simulink library "rewardLibrary"  (R2022b)
settings: Solver=VariableStepAuto  StartTime=0.0  StopTime=10.0  RelTol=1e-3
values from neighbouring files (symbols this model uses):
  accel_vec = (-4:0.5:4)'    [setUpModel.m]
  Ts = 0.1    [setUpMPC.m]
  TsRL = Ts    [setUpRLEnv.m]
  vel_vec = 0:2:20    [setUpModel.m]
undefined symbols (not defined in the file or in its folder): A, B, C, curvature1, D, D_default, DiscIntNeverNeededParam, E, F, gradbp1, k_sigmoid, steer_lim, t_gap, v_set, x_colpen, y_colpen, Z_colpen
libraries: simulink x379, $bdroot x2, mpcadaslib x1
(part 4 of 9)

== system rewardLibrary/Obs // Reward 2-3/Subsystem2 ==
  v_ego : Inport
  e1 : Inport  Port=2
  e2 : Inport  Port=3
  AND : Logic  IconShape=distinctive  AllPortsSameDT=off  OutDataTypeStr=boolean
  Abs : Abs  SaturateOnIntegerOverflow=off
  Abs1 : Abs  SaturateOnIntegerOverflow=off
  Lateral deviation : simulink/Logic and Bit Operations/Compare To Constant  relop=>  const=8  OutDataTypeStr=boolean
  Logical Operator : Logic  Operator=OR  AllPortsSameDT=off  OutDataTypeStr=boolean
  R2D : Gain  Gain=180/pi
  Relative yaw angle : simulink/Logic and Bit Operations/Compare To Constant  relop=>  const=60  OutDataTypeStr=boolean
  Velocity : simulink/Logic and Bit Operations/Compare To Constant  relop=<  const=0.5  OutDataTypeStr=boolean
  Velocity1 : simulink/Logic and Bit Operations/Compare To Constant  relop=<  const=10  OutDataTypeStr=boolean
  isDone : Outport  VectorParamsAs1DForOutWhenUnconnected=off
  spinTurn : Outport  Port=2  VectorParamsAs1DForOutWhenUnconnected=off
  wires:
  Velocity/1 -> Logical Operator/1
  Logical Operator/1 -> isDone/1
  v_ego/1 -> Velocity1/1, Velocity/1
  Abs/1 -> Lateral deviation/1
  Lateral deviation/1 -> Logical Operator/2
  e1/1 -> Abs/1
  Velocity1/1 -> AND/1
  e2/1 -> Abs1/1
  Abs1/1 -> R2D/1
  R2D/1 -> Relative yaw angle/1
  Relative yaw angle/1 -> AND/2
  AND/1 -> spinTurn/1

== system rewardLibrary/Obs // Reward 2-4/Subsystem ==
  v_ego : Inport
  v_ref : Inport  Port=2
  e1 : Inport  Port=3
  e2 : Inport  Port=4
  e1dot : Inport  Port=5
  e2dot : Inport  Port=6
  Add : Sum  Inputs=+-
  Discrete-Time Integrator1 : DiscreteIntegrator  SampleTime=-1  ICPrevOutput=DiscIntNeverNeededParam  ICPrevScaledInput=DiscIntNeverNeededParam
  Discrete-Time Integrator2 : DiscreteIntegrator  SampleTime=-1  ICPrevOutput=DiscIntNeverNeededParam  ICPrevScaledInput=DiscIntNeverNeededParam
  Discrete-Time Integrator3 : DiscreteIntegrator  SampleTime=-1  ICPrevOutput=DiscIntNeverNeededParam  ICPrevScaledInput=DiscIntNeverNeededParam
  Lateral deviation : Scope
  Mux : Mux  Inputs=9
  obs : Outport  VectorParamsAs1DForOutWhenUnconnected=off
  v_err : Outport  Port=2  VectorParamsAs1DForOutWhenUnconnected=off
  wires:
  Add/1 -> v_err/1, Mux/2, Discrete-Time Integrator1/1
  Discrete-Time Integrator3/1 -> Mux/6  "integral_error"
  v_ego/1 -> Add/2, Mux/3
  e1/1 -> Lateral deviation/1, Mux/5, Discrete-Time Integrator2/1
  Discrete-Time Integrator1/1 -> Mux/1  "integral_error"
  e2/1 -> Mux/7, Discrete-Time Integrator3/1
  Discrete-Time Integrator2/1 -> Mux/4  "integral_error"
  Mux/1 -> obs/1
  e1dot/1 -> Mux/8
  e2dot/1 -> Mux/9
  v_ref/1 -> Add/1  "d_rel"

== system rewardLibrary/Obs // Reward 2-4/Subsystem1 ==
  steer : Inport
  e1 : Inport  Port=2
  v_err : Inport  Port=3
  accel : Inport  Port=4
  Compare To Constant : simulink/Logic and Bit Operations/Compare To Constant  relop=<  const=1  OutDataTypeStr=boolean
  Compare To Constant1 : simulink/Logic and Bit Operations/Compare To Constant  relop=<  const=4  OutDataTypeStr=boolean
  Digital Clock : DigitalClock  Commented=on  SampleTime=Ts
  Gain : Gain  Gain=100
  Gain1 : Gain
  Gain2 : Gain  Gain=500
  Gain3 : Gain  Gain=2
  Gain4 : Gain  Gain=1e-3
  Gain5 : Gain  Commented=on  Gain=1/10
  Gain6 : Gain  Gain=100
  Gain7 : Gain  Gain=10
  Math Function2 : Math  Operator=square  SignedPower=on
  Square : Math  Operator=square  SignedPower=on
  Square2 : Math  Operator=square  SignedPower=on
  Square5 : Math  Operator=square  SignedPower=on
  Sum : Sum  Inputs=----
  Sum1 : Sum  Inputs=++++
  Unit Delay : UnitDelay  SampleTime=-1  HasFrameUpgradeWarning=on
  Unit Delay1 : UnitDelay  SampleTime=-1  HasFrameUpgradeWarning=on
  reward : Outport  VectorParamsAs1DForOutWhenUnconnected=off
  wires:
  v_err/1 -> Square5/1
  Square/1 -> Compare To Constant1/1, Gain/1
  Sum1/1 -> reward/1
  accel/1 -> Unit Delay1/1
  Gain6/1 -> Sum/4
  Compare To Constant/1 -> Gain1/1
  Math Function2/1 -> Gain6/1
  Gain3/1 -> Sum1/1
  Compare To Constant1/1 -> Gain3/1
  Square2/1 -> Gain2/1
  Gain7/1 -> Sum/3
  Unit Delay1/1 -> Math Function2/1
  Gain1/1 -> Sum1/3
  steer/1 -> Unit Delay/1
  Gain2/1 -> Sum/2
  Sum/1 -> Gain4/1
  Unit Delay/1 -> Square2/1
  Square5/1 -> Compare To Constant/1, Gain7/1
  Gain/1 -> Sum/1
  Gain4/1 -> Sum1/2
  e1/1 -> Square/1
  Digital Clock/1 -> Gain5/1
  Gain5/1 -> Sum1/4

== system rewardLibrary/Obs // Reward 2-4/Subsystem2 ==
  v_ego : Inport
  e1 : Inport  Port=2
  e2 : Inport  Port=3
  AND : Logic  IconShape=distinctive  AllPortsSameDT=off  OutDataTypeStr=boolean
  Abs : Abs  SaturateOnIntegerOverflow=off
  Abs1 : Abs  SaturateOnIntegerOverflow=off
  Lateral deviation : simulink/Logic and Bit Operations/Compare To Constant  relop=>  const=8  OutDataTypeStr=boolean
  Logical Operator : Logic  Operator=OR  AllPortsSameDT=off  OutDataTypeStr=boolean
  R2D : Gain  Gain=180/pi
  Relative yaw angle : simulink/Logic and Bit Operations/Compare To Constant  relop=>  const=60  OutDataTypeStr=boolean
  Velocity : simulink/Logic and Bit Operations/Compare To Constant  relop=<  const=0.5  OutDataTypeStr=boolean
  Velocity1 : simulink/Logic and Bit Operations/Compare To Constant  relop=<  const=10  OutDataTypeStr=boolean
  isDone : Outport  VectorParamsAs1DForOutWhenUnconnected=off
  spinTurn : Outport  Port=2  VectorParamsAs1DForOutWhenUnconnected=off
  wires:
  Velocity/1 -> Logical Operator/1
  Logical Operator/1 -> isDone/1
  v_ego/1 -> Velocity1/1, Velocity/1
  Abs/1 -> Lateral deviation/1
  Lateral deviation/1 -> Logical Operator/2
  e1/1 -> Abs/1
  Velocity1/1 -> AND/1
  e2/1 -> Abs1/1
  Abs1/1 -> R2D/1
  R2D/1 -> Relative yaw angle/1
  Relative yaw angle/1 -> AND/2
  AND/1 -> spinTurn/1

== system rewardLibrary/Obs // Reward 2-5/Subsystem ==
  v_ego : Inport
  v_ref : Inport  Port=2
  e1 : Inport  Port=3
  e2 : Inport  Port=4
  e1dot : Inport  Port=5
  e2dot : Inport  Port=6
  Add : Sum  Inputs=+-
  Discrete-Time Integrator1 : DiscreteIntegrator  SampleTime=-1  ICPrevOutput=DiscIntNeverNeededParam  ICPrevScaledInput=DiscIntNeverNeededParam
  Discrete-Time Integrator2 : DiscreteIntegrator  SampleTime=-1  ICPrevOutput=DiscIntNeverNeededParam  ICPrevScaledInput=DiscIntNeverNeededParam
  Discrete-Time Integrator3 : DiscreteIntegrator  SampleTime=-1  ICPrevOutput=DiscIntNeverNeededParam  ICPrevScaledInput=DiscIntNeverNeededParam
  Lateral deviation : Scope
  Mux : Mux  Inputs=9
  obs : Outport  VectorParamsAs1DForOutWhenUnconnected=off
  v_err : Outport  Port=2  VectorParamsAs1DForOutWhenUnconnected=off
  wires:
  Add/1 -> v_err/1, Mux/2, Discrete-Time Integrator1/1
  Discrete-Time Integrator3/1 -> Mux/6  "integral_error"
  v_ego/1 -> Add/2, Mux/3
  e1/1 -> Lateral deviation/1, Mux/5, Discrete-Time Integrator2/1
  Discrete-Time Integrator1/1 -> Mux/1  "integral_error"
  e2/1 -> Mux/7, Discrete-Time Integrator3/1
  Discrete-Time Integrator2/1 -> Mux/4  "integral_error"
  Mux/1 -> obs/1
  e1dot/1 -> Mux/8
  e2dot/1 -> Mux/9
  v_ref/1 -> Add/1  "d_rel"

== system rewardLibrary/Obs // Reward 2-5/Subsystem1 ==
  steer : Inport
  e1 : Inport  Port=2
  v_err : Inport  Port=3
  accel : Inport  Port=4
  Compare To Constant : simulink/Logic and Bit Operations/Compare To Constant  relop=<  const=1  OutDataTypeStr=boolean
  Compare To Constant1 : simulink/Logic and Bit Operations/Compare To Constant  relop=<  const=4  OutDataTypeStr=boolean
  Digital Clock : DigitalClock  Commented=on  SampleTime=Ts
  Gain : Gain  Gain=100
  Gain1 : Gain
  Gain2 : Gain  Gain=500
  Gain3 : Gain  Gain=2
  Gain4 : Gain  Gain=1e-3
  Gain5 : Gain  Commented=on  Gain=1/10
  Gain6 : Gain  Gain=100
  Gain7 : Gain  Gain=10
  Math Function2 : Math  Operator=square  SignedPower=on
  Square : Math  Operator=square  SignedPower=on
  Square2 : Math  Operator=square  SignedPower=on
  Square5 : Math  Operator=square  SignedPower=on
  Sum : Sum  Inputs=----
  Sum1 : Sum  Inputs=++++
  Unit Delay : UnitDelay  SampleTime=-1  HasFrameUpgradeWarning=on
  Unit Delay1 : UnitDelay  SampleTime=-1  HasFrameUpgradeWarning=on
  reward : Outport  VectorParamsAs1DForOutWhenUnconnected=off
  wires:
  v_err/1 -> Square5/1
  Square/1 -> Compare To Constant1/1, Gain/1
  Sum1/1 -> reward/1
  accel/1 -> Unit Delay1/1
  Gain6/1 -> Sum/4
  Compare To Constant/1 -> Gain1/1
  Math Function2/1 -> Gain6/1
  Gain3/1 -> Sum1/1
  Compare To Constant1/1 -> Gain3/1
  Square2/1 -> Gain2/1
  Gain7/1 -> Sum/3
  Unit Delay1/1 -> Math Function2/1
  Gain1/1 -> Sum1/3
  steer/1 -> Unit Delay/1
  Gain2/1 -> Sum/2
  Sum/1 -> Gain4/1
  Unit Delay/1 -> Square2/1
  Square5/1 -> Compare To Constant/1, Gain7/1
  Gain/1 -> Sum/1
  Gain4/1 -> Sum1/2
  e1/1 -> Square/1
  Digital Clock/1 -> Gain5/1
  Gain5/1 -> Sum1/4

== system rewardLibrary/Obs // Reward 2-5/Subsystem2 ==
  v_ego : Inport
  e1 : Inport  Port=2
  e2 : Inport  Port=3
  AND : Logic  IconShape=distinctive  AllPortsSameDT=off  OutDataTypeStr=boolean
  Abs : Abs  SaturateOnIntegerOverflow=off
  Abs1 : Abs  SaturateOnIntegerOverflow=off
  Lateral deviation : simulink/Logic and Bit Operations/Compare To Constant  relop=>  const=8  OutDataTypeStr=boolean
  Logical Operator : Logic  Operator=OR  AllPortsSameDT=off  OutDataTypeStr=boolean
  R2D : Gain  Gain=180/pi
  Relative yaw angle : simulink/Logic and Bit Operations/Compare To Constant  relop=>  const=60  OutDataTypeStr=boolean
  Velocity : simulink/Logic and Bit Operations/Compare To Constant  relop=<  const=2.5  OutDataTypeStr=boolean
  Velocity1 : simulink/Logic and Bit Operations/Compare To Constant  relop=<  const=10  OutDataTypeStr=boolean
  isDone : Outport  VectorParamsAs1DForOutWhenUnconnected=off
  spinTurn : Outport  Port=2  VectorParamsAs1DForOutWhenUnconnected=off
  wires:
  Velocity/1 -> Logical Operator/1
  Logical Operator/1 -> isDone/1
  v_ego/1 -> Velocity1/1, Velocity/1
  Abs/1 -> Lateral deviation/1
  Lateral deviation/1 -> Logical Operator/2
  e1/1 -> Abs/1
  Velocity1/1 -> AND/1
  e2/1 -> Abs1/1
  Abs1/1 -> R2D/1
  R2D/1 -> Relative yaw angle/1
  Relative yaw angle/1 -> AND/2
  AND/1 -> spinTurn/1

== system rewardLibrary/Obs // Reward 2-6/Subsystem ==
  v_ego : Inport
  v_ref : Inport  Port=2
  e1 : Inport  Port=3
  e2 : Inport  Port=4
  e1dot : Inport  Port=5
  e2dot : Inport  Port=6
  Add : Sum  Inputs=+-
  Discrete-Time Integrator1 : DiscreteIntegrator  SampleTime=-1  ICPrevOutput=DiscIntNeverNeededParam  ICPrevScaledInput=DiscIntNeverNeededParam
  Discrete-Time Integrator2 : DiscreteIntegrator  SampleTime=-1  ICPrevOutput=DiscIntNeverNeededParam  ICPrevScaledInput=DiscIntNeverNeededParam
  Discrete-Time Integrator3 : DiscreteIntegrator  SampleTime=-1  ICPrevOutput=DiscIntNeverNeededParam  ICPrevScaledInput=DiscIntNeverNeededParam
  Lateral deviation : Scope
  Mux : Mux  Inputs=9
  obs : Outport  VectorParamsAs1DForOutWhenUnconnected=off
  v_err : Outport  Port=2  VectorParamsAs1DForOutWhenUnconnected=off
  wires:
  Add/1 -> v_err/1, Mux/2, Discrete-Time Integrator1/1
  Discrete-Time Integrator3/1 -> Mux/6  "integral_error"
  v_ego/1 -> Add/2, Mux/3
  e1/1 -> Lateral deviation/1, Mux/5, Discrete-Time Integrator2/1
  Discrete-Time Integrator1/1 -> Mux/1  "integral_error"
  e2/1 -> Mux/7, Discrete-Time Integrator3/1
  Discrete-Time Integrator2/1 -> Mux/4  "integral_error"
  Mux/1 -> obs/1
  e1dot/1 -> Mux/8
  e2dot/1 -> Mux/9
  v_ref/1 -> Add/1  "d_rel"

== system rewardLibrary/Obs // Reward 2-6/Subsystem1 ==
  steer : Inport
  e1 : Inport  Port=2
  v_err : Inport  Port=3
  accel : Inport  Port=4
  Compare To Constant : simulink/Logic and Bit Operations/Compare To Constant  relop=<  const=1  OutDataTypeStr=boolean
  Compare To Constant1 : simulink/Logic and Bit Operations/Compare To Constant  relop=<  const=4  OutDataTypeStr=boolean
  Digital Clock : DigitalClock  Commented=on  SampleTime=Ts
  Gain : Gain  Gain=100
  Gain1 : Gain
  Gain2 : Gain  Gain=500
  Gain3 : Gain  Gain=2
  Gain4 : Gain  Gain=1e-3
  Gain5 : Gain  Commented=on  Gain=1/10
  Gain6 : Gain  Gain=100
  Gain7 : Gain  Gain=20
  Math Function2 : Math  Operator=square  SignedPower=on
  Square : Math  Operator=square  SignedPower=on
  Square2 : Math  Operator=square  SignedPower=on
  Square5 : Math  Operator=square  SignedPower=on
  Sum : Sum  Inputs=----
  Sum1 : Sum  Inputs=++++
  Unit Delay : UnitDelay  SampleTime=-1  HasFrameUpgradeWarning=on
  Unit Delay1 : UnitDelay  SampleTime=-1  HasFrameUpgradeWarning=on
  reward : Outport  VectorParamsAs1DForOutWhenUnconnected=off
  wires:
  v_err/1 -> Square5/1
  Square/1 -> Compare To Constant1/1, Gain/1
  Sum1/1 -> reward/1
  accel/1 -> Unit Delay1/1
  Gain6/1 -> Sum/4
  Compare To Constant/1 -> Gain1/1
  Math Function2/1 -> Gain6/1
  Gain3/1 -> Sum1/1
  Compare To Constant1/1 -> Gain3/1
  Square2/1 -> Gain2/1
  Gain7/1 -> Sum/3
  Unit Delay1/1 -> Math Function2/1
  Gain1/1 -> Sum1/3
  steer/1 -> Unit Delay/1
  Gain2/1 -> Sum/2
  Sum/1 -> Gain4/1
  Unit Delay/1 -> Square2/1
  Square5/1 -> Compare To Constant/1, Gain7/1
  Gain/1 -> Sum/1
  Gain4/1 -> Sum1/2
  e1/1 -> Square/1
  Digital Clock/1 -> Gain5/1
  Gain5/1 -> Sum1/4

== system rewardLibrary/Obs // Reward 2-6/Subsystem2 ==
  v_ego : Inport
  e1 : Inport  Port=2
  e2 : Inport  Port=3
  AND : Logic  IconShape=distinctive  AllPortsSameDT=off  OutDataTypeStr=boolean
  Abs : Abs  SaturateOnIntegerOverflow=off
  Abs1 : Abs  SaturateOnIntegerOverflow=off
  Lateral deviation : simulink/Logic and Bit Operations/Compare To Constant  relop=>  const=8  OutDataTypeStr=boolean
  Logical Operator : Logic  Operator=OR  AllPortsSameDT=off  OutDataTypeStr=boolean
  R2D : Gain  Gain=180/pi
  Relative yaw angle : simulink/Logic and Bit Operations/Compare To Constant  relop=>  const=60  OutDataTypeStr=boolean
  Velocity : simulink/Logic and Bit Operations/Compare To Constant  relop=<  const=4  OutDataTypeStr=boolean
  Velocity1 : simulink/Logic and Bit Operations/Compare To Constant  relop=<  const=10  OutDataTypeStr=boolean
  isDone : Outport  VectorParamsAs1DForOutWhenUnconnected=off
  spinTurn : Outport  Port=2  VectorParamsAs1DForOutWhenUnconnected=off
  wires:
  Velocity/1 -> Logical Operator/1
  Logical Operator/1 -> isDone/1
  v_ego/1 -> Velocity1/1, Velocity/1
  Abs/1 -> Lateral deviation/1
  Lateral deviation/1 -> Logical Operator/2
  e1/1 -> Abs/1
  Velocity1/1 -> AND/1
  e2/1 -> Abs1/1
  Abs1/1 -> R2D/1
  R2D/1 -> Relative yaw angle/1
  Relative yaw angle/1 -> AND/2
  AND/1 -> spinTurn/1

== system rewardLibrary/Obs // Reward 2-7/Subsystem ==
  v_ego : Inport
  v_ref : Inport  Port=2
  e1 : Inport  Port=3
  e2 : Inport  Port=4
  e1dot : Inport  Port=5
  e2dot : Inport  Port=6
  Add : Sum  Inputs=+-
  Discrete-Time Integrator1 : DiscreteIntegrator  SampleTime=-1  ICPrevOutput=DiscIntNeverNeededParam  ICPrevScaledInput=DiscIntNeverNeededParam
  Discrete-Time Integrator2 : DiscreteIntegrator  SampleTime=-1  ICPrevOutput=DiscIntNeverNeededParam  ICPrevScaledInput=DiscIntNeverNeededParam
  Discrete-Time Integrator3 : DiscreteIntegrator  SampleTime=-1  ICPrevOutput=DiscIntNeverNeededParam  ICPrevScaledInput=DiscIntNeverNeededParam
  Lateral deviation : Scope
  Mux : Mux  Inputs=9
  obs : Outport  VectorParamsAs1DForOutWhenUnconnected=off
  v_err : Outport  Port=2  VectorParamsAs1DForOutWhenUnconnected=off
  wires:
  Add/1 -> v_err/1, Mux/2, Discrete-Time Integrator1/1
  Discrete-Time Integrator3/1 -> Mux/6  "integral_error"
  v_ego/1 -> Add/2, Mux/3
  e1/1 -> Lateral deviation/1, Mux/5, Discrete-Time Integrator2/1
  Discrete-Time Integrator1/1 -> Mux/1  "integral_error"
  e2/1 -> Mux/7, Discrete-Time Integrator3/1
  Discrete-Time Integrator2/1 -> Mux/4  "integral_error"
  Mux/1 -> obs/1
  e1dot/1 -> Mux/8
  e2dot/1 -> Mux/9
  v_ref/1 -> Add/1  "d_rel"

== system rewardLibrary/Obs // Reward 2-7/Subsystem1 ==
  steer : Inport
  e1 : Inport  Port=2
  v_err : Inport  Port=3
  accel : Inport  Port=4
  Compare To Constant : simulink/Logic and Bit Operations/Compare To Constant  relop=<  const=1  OutDataTypeStr=boolean
  Compare To Constant1 : simulink/Logic and Bit Operations/Compare To Constant  relop=<  const=4  OutDataTypeStr=boolean
  Digital Clock : DigitalClock  Commented=on  SampleTime=Ts
  Gain : Gain  Gain=100
  Gain1 : Gain
  Gain2 : Gain  Gain=500
  Gain3 : Gain  Gain=2
  Gain4 : Gain  Gain=1e-3
  Gain5 : Gain  Commented=on  Gain=1/10
  Gain6 : Gain  Gain=100
  Gain7 : Gain  Gain=20
  Math Function2 : Math  Operator=square  SignedPower=on
  Square : Math  Operator=square  SignedPower=on
  Square2 : Math  Operator=square  SignedPower=on
  Square5 : Math  Operator=square  SignedPower=on
  Sum : Sum  Inputs=----
  Sum1 : Sum  Inputs=++++
  Unit Delay : UnitDelay  SampleTime=-1  HasFrameUpgradeWarning=on
  Unit Delay1 : UnitDelay  SampleTime=-1  HasFrameUpgradeWarning=on
  reward : Outport  VectorParamsAs1DForOutWhenUnconnected=off
  wires:
  v_err/1 -> Square5/1
  Square/1 -> Compare To Constant1/1, Gain/1
  Sum1/1 -> reward/1
  accel/1 -> Unit Delay1/1
  Gain6/1 -> Sum/4
  Compare To Constant/1 -> Gain1/1
  Math Function2/1 -> Gain6/1
  Gain3/1 -> Sum1/1
  Compare To Constant1/1 -> Gain3/1
  Square2/1 -> Gain2/1
  Gain7/1 -> Sum/3
  Unit Delay1/1 -> Math Function2/1
  Gain1/1 -> Sum1/3
  steer/1 -> Unit Delay/1
  Gain2/1 -> Sum/2
  Sum/1 -> Gain4/1
  Unit Delay/1 -> Square2/1
  Square5/1 -> Compare To Constant/1, Gain7/1
  Gain/1 -> Sum/1
  Gain4/1 -> Sum1/2
  e1/1 -> Square/1
  Digital Clock/1 -> Gain5/1
  Gain5/1 -> Sum1/4

== system rewardLibrary/Obs // Reward 2-7/Subsystem2 ==
  v_ego : Inport
  e1 : Inport  Port=2
  e2 : Inport  Port=3
  AND : Logic  IconShape=distinctive  AllPortsSameDT=off  OutDataTypeStr=boolean
  Abs : Abs  SaturateOnIntegerOverflow=off
  Abs1 : Abs  SaturateOnIntegerOverflow=off
  Lateral deviation : simulink/Logic and Bit Operations/Compare To Constant  relop=>  const=12  OutDataTypeStr=boolean
  Logical Operator : Logic  Operator=OR  AllPortsSameDT=off  OutDataTypeStr=boolean
  R2D : Gain  Gain=180/pi
  Relative yaw angle : simulink/Logic and Bit Operations/Compare To Constant  relop=>  const=60  OutDataTypeStr=boolean
  Velocity : simulink/Logic and Bit Operations/Compare To Constant  relop=<  const=4  OutDataTypeStr=boolean
  Velocity1 : simulink/Logic and Bit Operations/Compare To Constant  relop=<  const=10  OutDataTypeStr=boolean
  isDone : Outport  VectorParamsAs1DForOutWhenUnconnected=off
  spinTurn : Outport  Port=2  VectorParamsAs1DForOutWhenUnconnected=off
  wires:
  Velocity/1 -> Logical Operator/1
  Logical Operator/1 -> isDone/1
  v_ego/1 -> Velocity1/1, Velocity/1
  Abs/1 -> Lateral deviation/1
  Lateral deviation/1 -> Logical Operator/2
  e1/1 -> Abs/1
  Velocity1/1 -> AND/1
  e2/1 -> Abs1/1
  Abs1/1 -> R2D/1
  R2D/1 -> Relative yaw angle/1
  Relative yaw angle/1 -> AND/2
  AND/1 -> spinTurn/1

== system rewardLibrary/Obs // Reward 2-8/Subsystem ==
  v_ego : Inport
  v_ref : Inport  Port=2
  e1 : Inport  Port=3
  e2 : Inport  Port=4
  e1dot : Inport  Port=5
  e2dot : Inport  Port=6
  Add : Sum  Inputs=+-
  Discrete-Time Integrator1 : DiscreteIntegrator  SampleTime=-1  ICPrevOutput=DiscIntNeverNeededParam  ICPrevScaledInput=DiscIntNeverNeededParam
  Discrete-Time Integrator2 : DiscreteIntegrator  SampleTime=-1  ICPrevOutput=DiscIntNeverNeededParam  ICPrevScaledInput=DiscIntNeverNeededParam
  Discrete-Time Integrator3 : DiscreteIntegrator  SampleTime=-1  ICPrevOutput=DiscIntNeverNeededParam  ICPrevScaledInput=DiscIntNeverNeededParam
  Lateral deviation : Scope
  Mux : Mux  Inputs=9
  obs : Outport  VectorParamsAs1DForOutWhenUnconnected=off
  v_err : Outport  Port=2  VectorParamsAs1DForOutWhenUnconnected=off
  wires:
  Add/1 -> v_err/1, Mux/2, Discrete-Time Integrator1/1
  Discrete-Time Integrator3/1 -> Mux/6  "integral_error"
  v_ego/1 -> Add/2, Mux/3
  e1/1 -> Lateral deviation/1, Mux/5, Discrete-Time Integrator2/1
  Discrete-Time Integrator1/1 -> Mux/1  "integral_error"
  e2/1 -> Mux/7, Discrete-Time Integrator3/1
  Discrete-Time Integrator2/1 -> Mux/4  "integral_error"
  Mux/1 -> obs/1
  e1dot/1 -> Mux/8
  e2dot/1 -> Mux/9
  v_ref/1 -> Add/1  "d_rel"

== system rewardLibrary/Obs // Reward 2-8/Subsystem1 ==
  steer : Inport
  e1 : Inport  Port=2
  v_err : Inport  Port=3
  accel : Inport  Port=4
  Compare To Constant : simulink/Logic and Bit Operations/Compare To Constant  relop=<  const=1  OutDataTypeStr=boolean
  Compare To Constant1 : simulink/Logic and Bit Operations/Compare To Constant  relop=<  const=4  OutDataTypeStr=boolean
  Digital Clock : DigitalClock  Commented=on  SampleTime=Ts
  Gain : Gain  Gain=100
  Gain1 : Gain
  Gain2 : Gain  Gain=500
  Gain3 : Gain  Gain=2
  Gain4 : Gain  Gain=1e-3
  Gain5 : Gain  Commented=on  Gain=1/10
  Gain6 : Gain  Gain=100
  Gain7 : Gain  Gain=20
  Math Function2 : Math  Operator=square  SignedPower=on
  Square : Math  Operator=square  SignedPower=on
  Square2 : Math  Operator=square  SignedPower=on
  Square5 : Math  Operator=square  SignedPower=on
  Sum : Sum  Inputs=----
  Sum1 : Sum  Inputs=++++
  Unit Delay : UnitDelay  SampleTime=-1  HasFrameUpgradeWarning=on
  Unit Delay1 : UnitDelay  SampleTime=-1  HasFrameUpgradeWarning=on
  reward : Outport  VectorParamsAs1DForOutWhenUnconnected=off
  wires:
  v_err/1 -> Square5/1
  Square/1 -> Compare To Constant1/1, Gain/1
  Sum1/1 -> reward/1
  accel/1 -> Unit Delay1/1
  Gain6/1 -> Sum/4
  Compare To Constant/1 -> Gain1/1
  Math Function2/1 -> Gain6/1
  Gain3/1 -> Sum1/1
  Compare To Constant1/1 -> Gain3/1
  Square2/1 -> Gain2/1
  Gain7/1 -> Sum/3
  Unit Delay1/1 -> Math Function2/1
  Gain1/1 -> Sum1/3
  steer/1 -> Unit Delay/1
  Gain2/1 -> Sum/2
  Sum/1 -> Gain4/1
  Unit Delay/1 -> Square2/1
  Square5/1 -> Compare To Constant/1, Gain7/1
  Gain/1 -> Sum/1
  Gain4/1 -> Sum1/2
  e1/1 -> Square/1
  Digital Clock/1 -> Gain5/1
  Gain5/1 -> Sum1/4

== system rewardLibrary/Obs // Reward 2-8/Subsystem2 ==
  v_ego : Inport
  e1 : Inport  Port=2
  e2 : Inport  Port=3
  AND : Logic  IconShape=distinctive  AllPortsSameDT=off  OutDataTypeStr=boolean
  Abs : Abs  SaturateOnIntegerOverflow=off
  Abs1 : Abs  SaturateOnIntegerOverflow=off
  Lateral deviation : simulink/Logic and Bit Operations/Compare To Constant  relop=>  const=12  OutDataTypeStr=boolean
  Logical Operator : Logic  Operator=OR  AllPortsSameDT=off  OutDataTypeStr=boolean
  R2D : Gain  Gain=180/pi
  Relative yaw angle : simulink/Logic and Bit Operations/Compare To Constant  relop=>  const=60  OutDataTypeStr=boolean
  Velocity : simulink/Logic and Bit Operations/Compare To Constant  relop=<  const=4  OutDataTypeStr=boolean
  Velocity1 : simulink/Logic and Bit Operations/Compare To Constant  relop=<  const=10  OutDataTypeStr=boolean
  isDone : Outport  VectorParamsAs1DForOutWhenUnconnected=off
  spinTurn : Outport  Port=2  VectorParamsAs1DForOutWhenUnconnected=off
  wires:
  Velocity/1 -> Logical Operator/1
  Logical Operator/1 -> isDone/1
  v_ego/1 -> Velocity1/1, Velocity/1
  Abs/1 -> Lateral deviation/1
  Lateral deviation/1 -> Logical Operator/2
  e1/1 -> Abs/1
  Velocity1/1 -> AND/1
  e2/1 -> Abs1/1
  Abs1/1 -> R2D/1
  R2D/1 -> Relative yaw angle/1
  Relative yaw angle/1 -> AND/2
  AND/1 -> spinTurn/1

== system rewardLibrary/Obs // Reward 3-1/Subsystem ==
  v_ego : Inport
  v_ref : Inport  Port=2
  e1 : Inport  Port=3
  e2 : Inport  Port=4
  e1dot : Inport  Port=5
  e2dot : Inport  Port=6
  Add : Sum  Inputs=+-
  Discrete-Time Integrator1 : DiscreteIntegrator  SampleTime=-1  ICPrevOutput=DiscIntNeverNeededParam  ICPrevScaledInput=DiscIntNeverNeededParam
  Discrete-Time Integrator2 : DiscreteIntegrator  SampleTime=-1  ICPrevOutput=DiscIntNeverNeededParam  ICPrevScaledInput=DiscIntNeverNeededParam
  Discrete-Time Integrator3 : DiscreteIntegrator  SampleTime=-1  ICPrevOutput=DiscIntNeverNeededParam  ICPrevScaledInput=DiscIntNeverNeededParam
  Lateral deviation : Scope
  Mux : Mux  Inputs=9
  obs : Outport  VectorParamsAs1DForOutWhenUnconnected=off
  v_err : Outport  Port=2  VectorParamsAs1DForOutWhenUnconnected=off
  wires:
  Add/1 -> v_err/1, Mux/2, Discrete-Time Integrator1/1
  Discrete-Time Integrator3/1 -> Mux/6  "integral_error"
  v_ego/1 -> Add/2, Mux/3
  e1/1 -> Lateral deviation/1, Mux/5, Discrete-Time Integrator2/1
  Discrete-Time Integrator1/1 -> Mux/1  "integral_error"
  e2/1 -> Mux/7, Discrete-Time Integrator3/1
  Discrete-Time Integrator2/1 -> Mux/4  "integral_error"
  Mux/1 -> obs/1
  e1dot/1 -> Mux/8
  e2dot/1 -> Mux/9
  v_ref/1 -> Add/1  "d_rel"

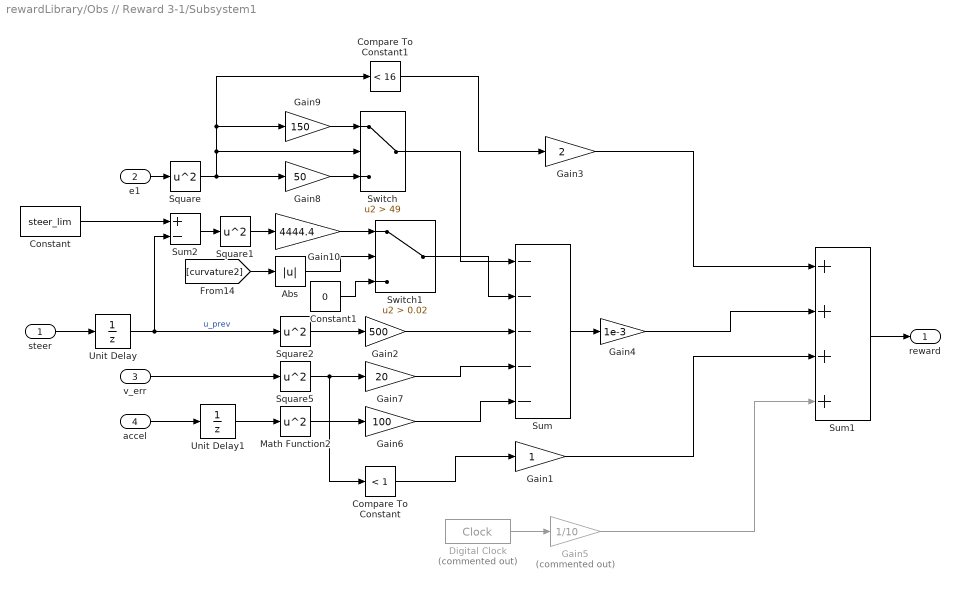
== system rewardLibrary/Obs // Reward 3-1/Subsystem1 ==
  steer : Inport
  e1 : Inport  Port=2
  v_err : Inport  Port=3
  accel : Inport  Port=4
  Abs : Abs  SaturateOnIntegerOverflow=off
  Compare To Constant : simulink/Logic and Bit Operations/Compare To Constant  relop=<  const=1  OutDataTypeStr=boolean
  Compare To Constant1 : simulink/Logic and Bit Operations/Compare To Constant  relop=<  const=16  OutDataTypeStr=boolean
  Constant : Constant  Value=steer_lim
  Constant1 : Constant  Value=0
  Digital Clock : DigitalClock  Commented=on  SampleTime=Ts
  Gain1 : Gain
  Gain10 : Gain  Gain=4444.4
  Gain2 : Gain  Gain=500
  Gain3 : Gain  Gain=2
  Gain4 : Gain  Gain=1e-3
  Gain5 : Gain  Commented=on  Gain=1/10
  Gain6 : Gain  Gain=100
  Gain7 : Gain  Gain=20
  Gain8 : Gain  Gain=50
  Gain9 : Gain  Gain=150
  Math Function2 : Math  Operator=square  SignedPower=on
  Square{,1..2,5} (4 alike) : Math  Operator=square  SignedPower=on
  Sum : Sum  Inputs=-----
  Sum1 : Sum  Inputs=++++
  Sum2 : Sum  Inputs=+-
  Switch : Switch  Criteria=u2 > Threshold  Threshold=49  SaturateOnIntegerOverflow=off  InputSameDT=off
  Switch1 : Switch  Criteria=u2 > Threshold  Threshold=0.02  SaturateOnIntegerOverflow=off  InputSameDT=off
  Unit Delay : UnitDelay  SampleTime=-1  HasFrameUpgradeWarning=on
  Unit Delay1 : UnitDelay  SampleTime=-1  HasFrameUpgradeWarning=on
  reward : Outport  VectorParamsAs1DForOutWhenUnconnected=off
  wires:
  v_err/1 -> Square5/1
  Square/1 -> Gain9/1, Compare To Constant1/1, Switch/2, Gain8/1
  Sum1/1 -> reward/1
  accel/1 -> Unit Delay1/1
  Gain6/1 -> Sum/5
  Compare To Constant/1 -> Gain1/1
  Math Function2/1 -> Gain6/1
  Gain3/1 -> Sum1/1
  Compare To Constant1/1 -> Gain3/1
  Square2/1 -> Gain2/1
  Gain7/1 -> Sum/4
  Unit Delay1/1 -> Math Function2/1
  Gain1/1 -> Sum1/3
  steer/1 -> Unit Delay/1
  Gain2/1 -> Sum/3
  Sum/1 -> Gain4/1
  Unit Delay/1 -> Square2/1, Sum2/2  "u_prev"
  Square5/1 -> Compare To Constant/1, Gain7/1
  Gain4/1 -> Sum1/2
  e1/1 -> Square/1
  Digital Clock/1 -> Gain5/1
  Gain5/1 -> Sum1/4
  Gain8/1 -> Switch/3
  Gain9/1 -> Switch/1
  Switch/1 -> Sum/1
  Constant/1 -> Sum2/1
  Sum2/1 -> Square1/1
  Square1/1 -> Gain10/1
  Gain10/1 -> Switch1/1
  [curvature2] -> Abs/1
  Abs/1 -> Switch1/2
  Switch1/1 -> Sum/2
  Constant1/1 -> Switch1/3

== system rewardLibrary/Obs // Reward 3-1/Subsystem2 ==
  v_ego : Inport
  e1 : Inport  Port=2
  e2 : Inport  Port=3
  AND : Logic  IconShape=distinctive  AllPortsSameDT=off  OutDataTypeStr=boolean
  Abs : Abs  SaturateOnIntegerOverflow=off
  Abs1 : Abs  SaturateOnIntegerOverflow=off
  Lateral deviation : simulink/Logic and Bit Operations/Compare To Constant  relop=>  const=12  OutDataTypeStr=boolean
  Logical Operator : Logic  Operator=OR  AllPortsSameDT=off  OutDataTypeStr=boolean
  R2D : Gain  Gain=180/pi
  Relative yaw angle : simulink/Logic and Bit Operations/Compare To Constant  relop=>  const=60  OutDataTypeStr=boolean
  Velocity : simulink/Logic and Bit Operations/Compare To Constant  relop=<  const=4  OutDataTypeStr=boolean
  Velocity1 : simulink/Logic and Bit Operations/Compare To Constant  relop=<  const=10  OutDataTypeStr=boolean
  isDone : Outport  VectorParamsAs1DForOutWhenUnconnected=off
  spinTurn : Outport  Port=2  VectorParamsAs1DForOutWhenUnconnected=off
  wires:
  Velocity/1 -> Logical Operator/1
  Logical Operator/1 -> isDone/1
  v_ego/1 -> Velocity1/1, Velocity/1
  Abs/1 -> Lateral deviation/1
  Lateral deviation/1 -> Logical Operator/2
  e1/1 -> Abs/1
  Velocity1/1 -> AND/1
  e2/1 -> Abs1/1
  Abs1/1 -> R2D/1
  R2D/1 -> Relative yaw angle/1
  Relative yaw angle/1 -> AND/2
  AND/1 -> spinTurn/1

== system rewardLibrary/Obs // Reward 3-2/Subsystem ==
  v_ego : Inport
  v_ref : Inport  Port=2
  e1 : Inport  Port=3
  e2 : Inport  Port=4
  e1dot : Inport  Port=5
  e2dot : Inport  Port=6
  Add : Sum  Inputs=+-
  Discrete-Time Integrator1 : DiscreteIntegrator  SampleTime=-1  ICPrevOutput=DiscIntNeverNeededParam  ICPrevScaledInput=DiscIntNeverNeededParam
  Discrete-Time Integrator2 : DiscreteIntegrator  SampleTime=-1  ICPrevOutput=DiscIntNeverNeededParam  ICPrevScaledInput=DiscIntNeverNeededParam
  Discrete-Time Integrator3 : DiscreteIntegrator  SampleTime=-1  ICPrevOutput=DiscIntNeverNeededParam  ICPrevScaledInput=DiscIntNeverNeededParam
  Lateral deviation : Scope
  Mux : Mux  Inputs=9
  obs : Outport  VectorParamsAs1DForOutWhenUnconnected=off
  v_err : Outport  Port=2  VectorParamsAs1DForOutWhenUnconnected=off
  wires:
  Add/1 -> v_err/1, Mux/2, Discrete-Time Integrator1/1
  Discrete-Time Integrator3/1 -> Mux/6  "integral_error"
  v_ego/1 -> Add/2, Mux/3
  e1/1 -> Lateral deviation/1, Mux/5, Discrete-Time Integrator2/1
  Discrete-Time Integrator1/1 -> Mux/1  "integral_error"
  e2/1 -> Mux/7, Discrete-Time Integrator3/1
  Discrete-Time Integrator2/1 -> Mux/4  "integral_error"
  Mux/1 -> obs/1
  e1dot/1 -> Mux/8
  e2dot/1 -> Mux/9
  v_ref/1 -> Add/1  "d_rel"

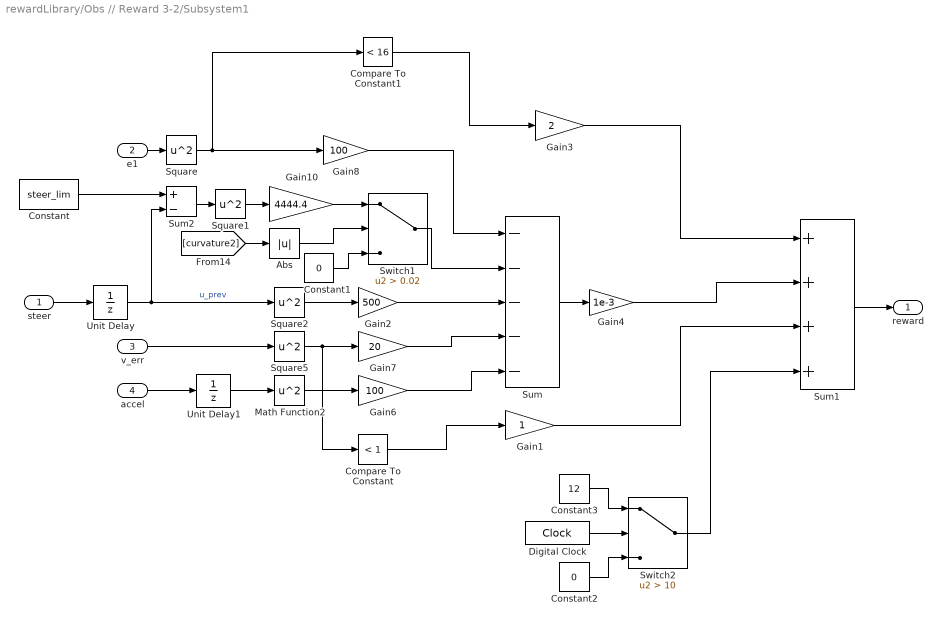
== system rewardLibrary/Obs // Reward 3-2/Subsystem1 ==
  steer : Inport
  e1 : Inport  Port=2
  v_err : Inport  Port=3
  accel : Inport  Port=4
  Abs : Abs  SaturateOnIntegerOverflow=off
  Compare To Constant : simulink/Logic and Bit Operations/Compare To Constant  relop=<  const=1  OutDataTypeStr=boolean
  Compare To Constant1 : simulink/Logic and Bit Operations/Compare To Constant  relop=<  const=16  OutDataTypeStr=boolean
  Constant : Constant  Value=steer_lim
  Constant1 : Constant  Value=0
  Constant2 : Constant  Value=0
  Constant3 : Constant  Value=12
  Digital Clock : DigitalClock  SampleTime=Ts
  Gain1 : Gain
  Gain10 : Gain  Gain=4444.4
  Gain2 : Gain  Gain=500
  Gain3 : Gain  Gain=2
  Gain4 : Gain  Gain=1e-3
  Gain6 : Gain  Gain=100
  Gain7 : Gain  Gain=20
  Gain8 : Gain  Gain=100
  Math Function2 : Math  Operator=square  SignedPower=on
  Square{,1..2,5} (4 alike) : Math  Operator=square  SignedPower=on
  Sum : Sum  Inputs=-----
  Sum1 : Sum  Inputs=++++
  Sum2 : Sum  Inputs=+-
  Switch1 : Switch  Criteria=u2 > Threshold  Threshold=0.02  SaturateOnIntegerOverflow=off  InputSameDT=off
  Switch2 : Switch  Criteria=u2 > Threshold  Threshold=10  SaturateOnIntegerOverflow=off  InputSameDT=off
  Unit Delay : UnitDelay  SampleTime=-1  HasFrameUpgradeWarning=on
  Unit Delay1 : UnitDelay  SampleTime=-1  HasFrameUpgradeWarning=on
  reward : Outport  VectorParamsAs1DForOutWhenUnconnected=off
  wires:
  v_err/1 -> Square5/1
  Square/1 -> Compare To Constant1/1, Gain8/1
  Sum1/1 -> reward/1
  accel/1 -> Unit Delay1/1
  Gain6/1 -> Sum/5
  Compare To Constant/1 -> Gain1/1
  Math Function2/1 -> Gain6/1
  Gain3/1 -> Sum1/1
  Compare To Constant1/1 -> Gain3/1
  Square2/1 -> Gain2/1
  Gain7/1 -> Sum/4
  Unit Delay1/1 -> Math Function2/1
  Gain1/1 -> Sum1/3
  steer/1 -> Unit Delay/1
  Gain2/1 -> Sum/3
  Sum/1 -> Gain4/1
  Unit Delay/1 -> Square2/1, Sum2/2  "u_prev"
  Square5/1 -> Compare To Constant/1, Gain7/1
  Gain4/1 -> Sum1/2
  e1/1 -> Square/1
  Digital Clock/1 -> Switch2/2
  Switch2/1 -> Sum1/4
  Gain8/1 -> Sum/1
  Constant/1 -> Sum2/1
  Sum2/1 -> Square1/1
  Square1/1 -> Gain10/1
  Gain10/1 -> Switch1/1
  [curvature2] -> Abs/1
  Abs/1 -> Switch1/2
  Switch1/1 -> Sum/2
  Constant1/1 -> Switch1/3
  Constant2/1 -> Switch2/3
  Constant3/1 -> Switch2/1

== system rewardLibrary/Obs // Reward 3-2/Subsystem2 ==
  v_ego : Inport
  e1 : Inport  Port=2
  e2 : Inport  Port=3
  AND : Logic  IconShape=distinctive  AllPortsSameDT=off  OutDataTypeStr=boolean
  Abs : Abs  SaturateOnIntegerOverflow=off
  Abs1 : Abs  SaturateOnIntegerOverflow=off
  Lateral deviation : simulink/Logic and Bit Operations/Compare To Constant  relop=>  const=12  OutDataTypeStr=boolean
  Logical Operator : Logic  Operator=OR  Inputs=3  AllPortsSameDT=off  OutDataTypeStr=boolean
  R2D : Gain  Gain=180/pi
  Relative yaw angle : simulink/Logic and Bit Operations/Compare To Constant  relop=>  const=60  OutDataTypeStr=boolean
  Velocity : simulink/Logic and Bit Operations/Compare To Constant  relop=<  const=4  OutDataTypeStr=boolean
  Velocity1 : simulink/Logic and Bit Operations/Compare To Constant  relop=<  const=10  OutDataTypeStr=boolean
  isDone : Outport  VectorParamsAs1DForOutWhenUnconnected=off
  wires:
  Velocity/1 -> Logical Operator/1
  Logical Operator/1 -> isDone/1
  v_ego/1 -> Velocity1/1, Velocity/1
  Abs/1 -> Lateral deviation/1
  Lateral deviation/1 -> Logical Operator/2
  e1/1 -> Abs/1
  Velocity1/1 -> AND/1
  e2/1 -> Abs1/1
  Abs1/1 -> R2D/1
  R2D/1 -> Relative yaw angle/1
  Relative yaw angle/1 -> AND/2
  AND/1 -> Logical Operator/3  "spinTurn"

== system rewardLibrary/Obs // Reward 3-3/Subsystem ==
  v_ego : Inport
  v_ref : Inport  Port=2
  e1 : Inport  Port=3
  e2 : Inport  Port=4
  e1dot : Inport  Port=5
  e2dot : Inport  Port=6
  Add : Sum  Inputs=+-
  Discrete-Time Integrator1 : DiscreteIntegrator  SampleTime=-1  ICPrevOutput=DiscIntNeverNeededParam  ICPrevScaledInput=DiscIntNeverNeededParam
  Discrete-Time Integrator2 : DiscreteIntegrator  SampleTime=-1  ICPrevOutput=DiscIntNeverNeededParam  ICPrevScaledInput=DiscIntNeverNeededParam
  Discrete-Time Integrator3 : DiscreteIntegrator  SampleTime=-1  ICPrevOutput=DiscIntNeverNeededParam  ICPrevScaledInput=DiscIntNeverNeededParam
  Lateral deviation : Scope
  Mux : Mux  Inputs=9
  obs : Outport  VectorParamsAs1DForOutWhenUnconnected=off
  v_err : Outport  Port=2  VectorParamsAs1DForOutWhenUnconnected=off
  wires:
  Add/1 -> v_err/1, Mux/2, Discrete-Time Integrator1/1
  Discrete-Time Integrator3/1 -> Mux/6  "integral_error"
  v_ego/1 -> Add/2, Mux/3
  e1/1 -> Lateral deviation/1, Mux/5, Discrete-Time Integrator2/1
  Discrete-Time Integrator1/1 -> Mux/1  "integral_error"
  e2/1 -> Mux/7, Discrete-Time Integrator3/1
  Discrete-Time Integrator2/1 -> Mux/4  "integral_error"
  Mux/1 -> obs/1
  e1dot/1 -> Mux/8
  e2dot/1 -> Mux/9
  v_ref/1 -> Add/1  "d_rel"

== system rewardLibrary/Obs // Reward 3-3/Subsystem1 ==
  steer : Inport
  e1 : Inport  Port=2
  v_err : Inport  Port=3
  accel : Inport  Port=4
  Compare To Constant : simulink/Logic and Bit Operations/Compare To Constant  relop=<  const=1  OutDataTypeStr=boolean
  Compare To Constant1 : simulink/Logic and Bit Operations/Compare To Constant  relop=<  const=16  OutDataTypeStr=boolean
  Constant2 : Constant  Value=0
  Constant3 : Constant  Value=12
  Digital Clock : DigitalClock  SampleTime=Ts
  Gain1 : Gain
  Gain2 : Gain  Gain=500
  Gain3 : Gain  Gain=2
  Gain4 : Gain  Gain=1e-3
  Gain6 : Gain  Gain=100
  Gain7 : Gain  Gain=20
  Gain8 : Gain  Gain=100
  Math Function2 : Math  Operator=square  SignedPower=on
  Square : Math  Operator=square  SignedPower=on
  Square2 : Math  Operator=square  SignedPower=on
  Square5 : Math  Operator=square  SignedPower=on
  Sum : Sum  Inputs=-----
  Sum1 : Sum  Inputs=++++
  Switch2 : Switch  Criteria=u2 > Threshold  Threshold=10  SaturateOnIntegerOverflow=off  InputSameDT=off
  Unit Delay : UnitDelay  SampleTime=-1  HasFrameUpgradeWarning=on
  Unit Delay1 : UnitDelay  SampleTime=-1  HasFrameUpgradeWarning=on
  turn assist : Subsystem  Commented=on
  reward : Outport  VectorParamsAs1DForOutWhenUnconnected=off
  wires:
  v_err/1 -> Square5/1
  Square/1 -> Compare To Constant1/1, Gain8/1
  Sum1/1 -> reward/1
  accel/1 -> Unit Delay1/1
  Gain6/1 -> Sum/5
  Compare To Constant/1 -> Gain1/1
  Math Function2/1 -> Gain6/1
  Gain3/1 -> Sum1/1
  Compare To Constant1/1 -> Gain3/1
  Square2/1 -> Gain2/1
  Gain7/1 -> Sum/4
  Unit Delay1/1 -> Math Function2/1
  Gain1/1 -> Sum1/3
  steer/1 -> Unit Delay/1
  Gain2/1 -> Sum/3
  Sum/1 -> Gain4/1
  Unit Delay/1 -> turn assist/1(u_prev), Square2/1  "u_prev"
  Square5/1 -> Compare To Constant/1, Gain7/1
  Gain4/1 -> Sum1/2
  e1/1 -> Square/1
  Digital Clock/1 -> Switch2/2
  Switch2/1 -> Sum1/4
  Gain8/1 -> Sum/1
  Constant2/1 -> Switch2/3
  Constant3/1 -> Switch2/1
  turn assist/1(Out1) -> Sum/2

== system rewardLibrary/Obs // Reward 3-3/Subsystem2 ==
  v_ego : Inport
  e1 : Inport  Port=2
  e2 : Inport  Port=3
  AND : Logic  IconShape=distinctive  AllPortsSameDT=off  OutDataTypeStr=boolean
  Abs : Abs  SaturateOnIntegerOverflow=off
  Abs1 : Abs  SaturateOnIntegerOverflow=off
  Lateral deviation : simulink/Logic and Bit Operations/Compare To Constant  relop=>  const=12  OutDataTypeStr=boolean
  Logical Operator : Logic  Operator=OR  Inputs=3  AllPortsSameDT=off  OutDataTypeStr=boolean
  R2D : Gain  Gain=180/pi
  Relative yaw angle : simulink/Logic and Bit Operations/Compare To Constant  relop=>  const=60  OutDataTypeStr=boolean
  Velocity : simulink/Logic and Bit Operations/Compare To Constant  relop=<  const=4  OutDataTypeStr=boolean
  Velocity1 : simulink/Logic and Bit Operations/Compare To Constant  relop=<  const=10  OutDataTypeStr=boolean
  isDone : Outport  VectorParamsAs1DForOutWhenUnconnected=off
  wires:
  Velocity/1 -> Logical Operator/1
  Logical Operator/1 -> isDone/1
  v_ego/1 -> Velocity1/1, Velocity/1
  Abs/1 -> Lateral deviation/1
  Lateral deviation/1 -> Logical Operator/2
  e1/1 -> Abs/1
  Velocity1/1 -> AND/1
  e2/1 -> Abs1/1
  Abs1/1 -> R2D/1
  R2D/1 -> Relative yaw angle/1
  Relative yaw angle/1 -> AND/2
  AND/1 -> Logical Operator/3  "spinTurn"

== system rewardLibrary/Obs // Reward 3-4/Subsystem ==
  v_ego : Inport
  v_ref : Inport  Port=2
  e1 : Inport  Port=3
  e2 : Inport  Port=4
  e1dot : Inport  Port=5
  e2dot : Inport  Port=6
  Add : Sum  Inputs=+-
  Discrete-Time Integrator1 : DiscreteIntegrator  SampleTime=-1  ICPrevOutput=DiscIntNeverNeededParam  ICPrevScaledInput=DiscIntNeverNeededParam
  Discrete-Time Integrator2 : DiscreteIntegrator  SampleTime=-1  ICPrevOutput=DiscIntNeverNeededParam  ICPrevScaledInput=DiscIntNeverNeededParam
  Discrete-Time Integrator3 : DiscreteIntegrator  SampleTime=-1  ICPrevOutput=DiscIntNeverNeededParam  ICPrevScaledInput=DiscIntNeverNeededParam
  Lateral deviation : Scope
  Mux : Mux  Inputs=9
  obs : Outport  VectorParamsAs1DForOutWhenUnconnected=off
  v_err : Outport  Port=2  VectorParamsAs1DForOutWhenUnconnected=off
  wires:
  Add/1 -> v_err/1, Mux/2, Discrete-Time Integrator1/1
  Discrete-Time Integrator3/1 -> Mux/6  "integral_error"
  v_ego/1 -> Add/2, Mux/3
  e1/1 -> Lateral deviation/1, Mux/5, Discrete-Time Integrator2/1
  Discrete-Time Integrator1/1 -> Mux/1  "integral_error"
  e2/1 -> Mux/7, Discrete-Time Integrator3/1
  Discrete-Time Integrator2/1 -> Mux/4  "integral_error"
  Mux/1 -> obs/1
  e1dot/1 -> Mux/8
  e2dot/1 -> Mux/9
  v_ref/1 -> Add/1  "d_rel"

== system rewardLibrary/Obs // Reward 3-4/Subsystem1 ==
  steer : Inport
  e1 : Inport  Port=2
  v_err : Inport  Port=3
  accel : Inport  Port=4
  Compare To Constant : simulink/Logic and Bit Operations/Compare To Constant  relop=<  const=1  OutDataTypeStr=boolean
  Compare To Constant1 : simulink/Logic and Bit Operations/Compare To Constant  relop=<  const=16  OutDataTypeStr=boolean
  Constant2 : Constant  Value=0
  Constant3 : Constant  Value=12
  Digital Clock : DigitalClock  SampleTime=Ts
  Gain1 : Gain
  Gain2 : Gain  Gain=500
  Gain3 : Gain  Gain=2
  Gain4 : Gain  Gain=1e-3
  Gain6 : Gain  Gain=100
  Gain7 : Gain  Gain=20
  Gain8 : Gain  Gain=100
  Math Function2 : Math  Operator=square  SignedPower=on
  Square : Math  Operator=square  SignedPower=on
  Square2 : Math  Operator=square  SignedPower=on
  Square5 : Math  Operator=square  SignedPower=on
  Sum : Sum  Inputs=-----
  Sum1 : Sum  Inputs=++++
  Switch2 : Switch  Criteria=u2 > Threshold  Threshold=10  SaturateOnIntegerOverflow=off  InputSameDT=off
  Unit Delay : UnitDelay  SampleTime=-1  HasFrameUpgradeWarning=on
  Unit Delay1 : UnitDelay  SampleTime=-1  HasFrameUpgradeWarning=on
  turn assist : Subsystem  Commented=on
  reward : Outport  VectorParamsAs1DForOutWhenUnconnected=off
  wires:
  v_err/1 -> Square5/1
  Square/1 -> Compare To Constant1/1, Gain8/1
  Sum1/1 -> reward/1
  accel/1 -> Unit Delay1/1
  Gain6/1 -> Sum/5
  Compare To Constant/1 -> Gain1/1
  Math Function2/1 -> Gain6/1
  Gain3/1 -> Sum1/1
  Compare To Constant1/1 -> Gain3/1
  Square2/1 -> Gain2/1
  Gain7/1 -> Sum/4
  Unit Delay1/1 -> Math Function2/1
  Gain1/1 -> Sum1/3
  steer/1 -> Unit Delay/1
  Gain2/1 -> Sum/3
  Sum/1 -> Gain4/1
  Unit Delay/1 -> turn assist/1(u_prev), Square2/1  "u_prev"
  Square5/1 -> Compare To Constant/1, Gain7/1
  Gain4/1 -> Sum1/2
  e1/1 -> Square/1
  Digital Clock/1 -> Switch2/2
  Switch2/1 -> Sum1/4
  Gain8/1 -> Sum/1
  Constant2/1 -> Switch2/3
  Constant3/1 -> Switch2/1
  turn assist/1(Out1) -> Sum/2

== system rewardLibrary/Obs // Reward 3-4/Subsystem2 ==
  v_ego : Inport
  e1 : Inport  Port=2
  e2 : Inport  Port=3
  AND : Logic  IconShape=distinctive  AllPortsSameDT=off  OutDataTypeStr=boolean
  Abs : Abs  SaturateOnIntegerOverflow=off
  Abs1 : Abs  SaturateOnIntegerOverflow=off
  Lateral deviation : simulink/Logic and Bit Operations/Compare To Constant  relop=>  const=12  OutDataTypeStr=boolean
  Logical Operator : Logic  Operator=OR  AllPortsSameDT=off  OutDataTypeStr=boolean
  R2D : Gain  Gain=180/pi
  Relative yaw angle : simulink/Logic and Bit Operations/Compare To Constant  relop=>  const=60  OutDataTypeStr=boolean
  Velocity : simulink/Logic and Bit Operations/Compare To Constant  relop=<  const=4  OutDataTypeStr=boolean
  Velocity1 : simulink/Logic and Bit Operations/Compare To Constant  relop=<  const=10  OutDataTypeStr=boolean
  isDone : Outport  VectorParamsAs1DForOutWhenUnconnected=off
  spinTurn : Outport  Port=2  VectorParamsAs1DForOutWhenUnconnected=off
  wires:
  Velocity/1 -> Logical Operator/1
  Logical Operator/1 -> isDone/1
  v_ego/1 -> Velocity1/1, Velocity/1
  Abs/1 -> Lateral deviation/1
  Lateral deviation/1 -> Logical Operator/2
  e1/1 -> Abs/1
  Velocity1/1 -> AND/1
  e2/1 -> Abs1/1
  Abs1/1 -> R2D/1
  R2D/1 -> Relative yaw angle/1
  Relative yaw angle/1 -> AND/2
  AND/1 -> spinTurn/1  "spinTurn"

== system rewardLibrary/Obs // Reward 3-5/Subsystem ==
  v_ego : Inport
  v_ref : Inport  Port=2
  e1 : Inport  Port=3
  e2 : Inport  Port=4
  e1dot : Inport  Port=5
  e2dot : Inport  Port=6
  Add : Sum  Inputs=+-
  Discrete-Time Integrator1 : DiscreteIntegrator  SampleTime=-1  ICPrevOutput=DiscIntNeverNeededParam  ICPrevScaledInput=DiscIntNeverNeededParam
  Discrete-Time Integrator2 : DiscreteIntegrator  SampleTime=-1  ICPrevOutput=DiscIntNeverNeededParam  ICPrevScaledInput=DiscIntNeverNeededParam
  Discrete-Time Integrator3 : DiscreteIntegrator  SampleTime=-1  ICPrevOutput=DiscIntNeverNeededParam  ICPrevScaledInput=DiscIntNeverNeededParam
  Lateral deviation : Scope
  Mux : Mux  Inputs=9
  obs : Outport  VectorParamsAs1DForOutWhenUnconnected=off
  v_err : Outport  Port=2  VectorParamsAs1DForOutWhenUnconnected=off
  wires:
  Add/1 -> v_err/1, Mux/2, Discrete-Time Integrator1/1
  Discrete-Time Integrator3/1 -> Mux/6  "integral_error"
  v_ego/1 -> Add/2, Mux/3
  e1/1 -> Lateral deviation/1, Mux/5, Discrete-Time Integrator2/1
  Discrete-Time Integrator1/1 -> Mux/1  "integral_error"
  e2/1 -> Mux/7, Discrete-Time Integrator3/1
  Discrete-Time Integrator2/1 -> Mux/4  "integral_error"
  Mux/1 -> obs/1
  e1dot/1 -> Mux/8
  e2dot/1 -> Mux/9
  v_ref/1 -> Add/1  "d_rel"

== system rewardLibrary/Obs // Reward 3-5/Subsystem1 ==
  steer : Inport
  e1 : Inport  Port=2
  v_err : Inport  Port=3
  accel : Inport  Port=4
  Compare To Constant : simulink/Logic and Bit Operations/Compare To Constant  relop=<  const=1  OutDataTypeStr=boolean
  Compare To Constant1 : simulink/Logic and Bit Operations/Compare To Constant  relop=<  const=16  OutDataTypeStr=boolean
  Constant2 : Constant  Value=0
  Constant3 : Constant  Value=2.2
  Digital Clock : DigitalClock  SampleTime=Ts
  Gain1 : Gain
  Gain2 : Gain  Gain=500
  Gain3 : Gain  Gain=2
  Gain4 : Gain  Gain=1e-3
  Gain6 : Gain  Gain=100
  Gain7 : Gain  Gain=20
  Gain8 : Gain  Gain=100
  Math Function2 : Math  Operator=square  SignedPower=on
  Square : Math  Operator=square  SignedPower=on
  Square2 : Math  Operator=square  SignedPower=on
  Square5 : Math  Operator=square  SignedPower=on
  Sum : Sum  Inputs=-----
  Sum1 : Sum  Inputs=++++
  Switch2 : Switch  Criteria=u2 > Threshold  Threshold=10  SaturateOnIntegerOverflow=off  InputSameDT=off
  Unit Delay : UnitDelay  SampleTime=-1  HasFrameUpgradeWarning=on
  Unit Delay1 : UnitDelay  SampleTime=-1  HasFrameUpgradeWarning=on
  turn assist : Subsystem  Commented=on
  reward : Outport  VectorParamsAs1DForOutWhenUnconnected=off
  wires:
  v_err/1 -> Square5/1
  Square/1 -> Compare To Constant1/1, Gain8/1
  Sum1/1 -> reward/1
  accel/1 -> Unit Delay1/1
  Gain6/1 -> Sum/5
  Compare To Constant/1 -> Gain1/1
  Math Function2/1 -> Gain6/1
  Gain3/1 -> Sum1/1
  Compare To Constant1/1 -> Gain3/1
  Square2/1 -> Gain2/1
  Gain7/1 -> Sum/4
  Unit Delay1/1 -> Math Function2/1
  Gain1/1 -> Sum1/3
  steer/1 -> Unit Delay/1
  Gain2/1 -> Sum/3
  Sum/1 -> Gain4/1
  Unit Delay/1 -> turn assist/1(u_prev), Square2/1  "u_prev"
  Square5/1 -> Compare To Constant/1, Gain7/1
  Gain4/1 -> Sum1/2
  e1/1 -> Square/1
  Digital Clock/1 -> Switch2/2
  Switch2/1 -> Sum1/4
  Gain8/1 -> Sum/1
  Constant2/1 -> Switch2/3
  Constant3/1 -> Switch2/1
  turn assist/1(Out1) -> Sum/2

== system rewardLibrary/Obs // Reward 3-5/Subsystem2 ==
  v_ego : Inport
  e1 : Inport  Port=2
  e2 : Inport  Port=3
  AND : Logic  IconShape=distinctive  AllPortsSameDT=off  OutDataTypeStr=boolean
  Abs : Abs  SaturateOnIntegerOverflow=off
  Abs1 : Abs  SaturateOnIntegerOverflow=off
  Lateral deviation : simulink/Logic and Bit Operations/Compare To Constant  relop=>  const=12  OutDataTypeStr=boolean
  Logical Operator : Logic  Operator=OR  AllPortsSameDT=off  OutDataTypeStr=boolean
  R2D : Gain  Gain=180/pi
  Relative yaw angle : simulink/Logic and Bit Operations/Compare To Constant  relop=>  const=55  OutDataTypeStr=boolean
  Velocity : simulink/Logic and Bit Operations/Compare To Constant  relop=<  const=2  OutDataTypeStr=boolean
  Velocity1 : simulink/Logic and Bit Operations/Compare To Constant  relop=<  const=5  OutDataTypeStr=boolean
  isDone : Outport  VectorParamsAs1DForOutWhenUnconnected=off
  spinTurn : Outport  Port=2  VectorParamsAs1DForOutWhenUnconnected=off
  wires:
  Velocity/1 -> Logical Operator/1
  Logical Operator/1 -> isDone/1
  v_ego/1 -> Velocity1/1, Velocity/1
  Abs/1 -> Lateral deviation/1
  Lateral deviation/1 -> Logical Operator/2
  e1/1 -> Abs/1
  Velocity1/1 -> AND/1
  e2/1 -> Abs1/1
  Abs1/1 -> R2D/1
  R2D/1 -> Relative yaw angle/1
  Relative yaw angle/1 -> AND/2
  AND/1 -> spinTurn/1  "spinTurn"

== system rewardLibrary/Obs // Reward 3-6/Subsystem ==
  v_ego : Inport
  v_ref : Inport  Port=2
  e1 : Inport  Port=3
  e2 : Inport  Port=4
  e1dot : Inport  Port=5
  e2dot : Inport  Port=6
  Add : Sum  Inputs=+-
  Discrete-Time Integrator1 : DiscreteIntegrator  SampleTime=-1  ICPrevOutput=DiscIntNeverNeededParam  ICPrevScaledInput=DiscIntNeverNeededParam
  Discrete-Time Integrator2 : DiscreteIntegrator  SampleTime=-1  ICPrevOutput=DiscIntNeverNeededParam  ICPrevScaledInput=DiscIntNeverNeededParam
  Discrete-Time Integrator3 : DiscreteIntegrator  SampleTime=-1  ICPrevOutput=DiscIntNeverNeededParam  ICPrevScaledInput=DiscIntNeverNeededParam
  Lateral deviation : Scope
  Mux : Mux  Inputs=9
  obs : Outport  VectorParamsAs1DForOutWhenUnconnected=off
  v_err : Outport  Port=2  VectorParamsAs1DForOutWhenUnconnected=off
  wires:
  Add/1 -> v_err/1, Mux/2, Discrete-Time Integrator1/1
  Discrete-Time Integrator3/1 -> Mux/6  "integral_error"
  v_ego/1 -> Add/2, Mux/3
  e1/1 -> Lateral deviation/1, Mux/5, Discrete-Time Integrator2/1
  Discrete-Time Integrator1/1 -> Mux/1  "integral_error"
  e2/1 -> Mux/7, Discrete-Time Integrator3/1
  Discrete-Time Integrator2/1 -> Mux/4  "integral_error"
  Mux/1 -> obs/1
  e1dot/1 -> Mux/8
  e2dot/1 -> Mux/9
  v_ref/1 -> Add/1  "d_rel"
